simulink model "bldc_motor2"  (Simulink 8.4)
settings: Solver=ode45  StartTime=0.0  StopTime=1  MaxStep=1e-4  RelTol=1e-4  AbsTol=1e-4
values from neighbouring files (symbols this model uses):
  Dm = 6.04e-6    (= 6.04e-06)    [bldc_par.m]
  J = 2.12e-6    (= 2.12e-06)    [bldc_par.m]
  Lam = 0.0165    [bldc_par.m]
  Lss = 10.1e-3    (= 0.0101)    [bldc_par.m]
  P = 2    [bldc_par.m]
  rs = 5.2    [bldc_par.m]
  Tm = 3.53e-3    (= 0.00353)    [bldc_par.m]
  Ts = Lss/rs    (= 0.00194230769231)    [bldc_par.m]
  Vdc = 6    [bldc_par.m]
undefined symbols (not defined in the file or in its folder): sgn
settings Model: Creator=Kevin Ta  LastModifiedBy=Kevin Ta
settings DataIOCC: MaxDataPoints=10000  SaveOutput=off  SaveState=on  StateSaveName=x  TimeSaveName=t  SignalLoggingName=sigsOut
settings OptimizationCC: ExpressionDepthLimit=128  InitFltsAndDblsToZero=on
settings DebuggingCC: SaveWithParameterizedLinksMsg=none  SignalResolutionControl=TryResolveAllWithWarning  SolverPrmCheckMsg=none  MultiTaskDSMMsg=warning  MultiTaskCondExecSysMsg=none  StateNameClashWarn=none
settings HardwareCC: TargetUnknown=on
settings RTWCC: IncludeERTFirstTime=on
settings GRTTargetCC: TargetFcnLib=ansi_tfl_tmw.mat

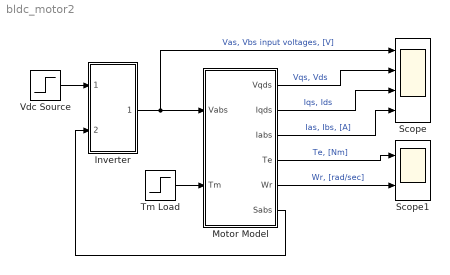
== system bldc_motor2 ==
  Inverter : Subsystem
  Motor Model : Subsystem
  Scope : Scope  NumInputPorts=4
      settings: TimeRange=1  YMin=-10~-10~-1~-1  YMax=10~10~2~2
  Scope1 : Scope  NumInputPorts=2
      settings: TimeRange=1  YMin=0~0  YMax=0.025~400
  Tm Load : Step  Time=0.5  After=Tm  SampleTime=0
  Vdc Source : Step  Time=0.05  After=Vdc  SampleTime=0
  wires:
  Inverter/1(Vabs) -> Scope/1, Motor Model/1(Vabs)  "Vas, Vbs input voltages, [V]"
  Vdc Source/1 -> Inverter/1(Vdc)
  Motor Model/1(Vqds) -> Scope/2  "Vqs, Vds"
  Motor Model/2(Iqds) -> Scope/3  "Iqs, Ids"
  Motor Model/3(Iabs) -> Scope/4  "Ias, Ibs, [A]"
  Motor Model/4(Te) -> Scope1/1  "Te, [Nm]"
  Motor Model/5(Wr) -> Scope1/2  "Wr, [rad/sec]"
  Tm Load/1 -> Motor Model/2(Tm)
  Motor Model/6(Sabs) -> Inverter/2(Sabs)

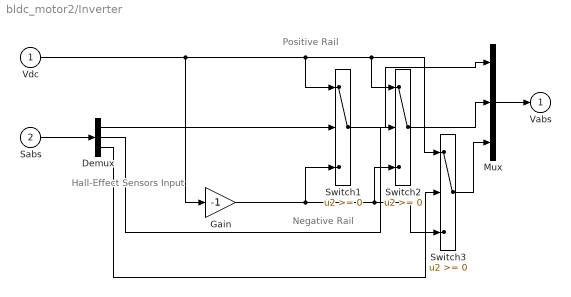
== system bldc_motor2/Inverter ==
  note: Positive Rail
  note: Negative Rail
  note: Hall-Effect
      | Sensors
      | Input
  Vdc : Inport
  Sabs : Inport  Port=2
  Demux : Demux  Outputs=3
  Gain : Gain  Gain=-1  SaturateOnIntegerOverflow=on  OutDataTypeStr=Inherit: Same as input  ParamDataTypeStr=Inherit: Same as input
  Mux : Mux  Inputs=3
  Switch1 : Switch  SaturateOnIntegerOverflow=on
  Switch2 : Switch  SaturateOnIntegerOverflow=on
  Switch3 : Switch  SaturateOnIntegerOverflow=on
  Vabs : Outport  InitialOutput=0
  wires:
  Vdc/1 -> Switch1/1, Switch3/1, Switch2/1, Gain/1
  Gain/1 -> Switch1/3, Switch3/3, Switch2/3
  Switch1/1 -> Mux/1
  Switch2/1 -> Mux/2
  Mux/1 -> Vabs/1
  Sabs/1 -> Demux/1
  Demux/1 -> Switch1/2
  Demux/2 -> Switch2/2
  Demux/3 -> Switch3/2
  Switch3/1 -> Mux/3

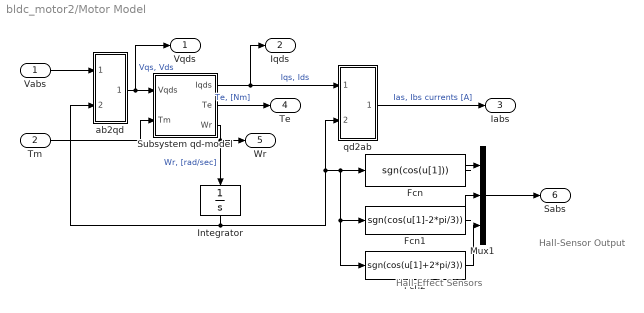
== system bldc_motor2/Motor Model ==
  note: Hall-Effect
      | Sensors
  note: Hall-Sensor
      | Output
  Vabs : Inport
  Tm : Inport  Port=2
  Fcn : Fcn  Expr=sgn(cos(u[1]))
  Fcn1 : Fcn  Expr=sgn(cos(u[1]-2*pi/3))
  Fcn2 : Fcn  Expr=sgn(cos(u[1]+2*pi/3))
  Integrator : Integrator
  Mux1 : Mux  Inputs=3
  Subsystem qd-model : Subsystem
  ab2qd : Subsystem
  qd2ab : Subsystem
  Vqds : Outport
  Iqds : Outport  Port=2
  Iabs : Outport  Port=3
  Te : Outport  Port=4
  Wr : Outport  Port=5
  Sabs : Outport  Port=6
  wires:
  ab2qd/1(Vqds) -> Subsystem qd-model/1(Vqds), Vqds/1  "Vqs, Vds"
  Subsystem qd-model/1(Iqds) -> qd2ab/1(Iqds), Iqds/1  "Iqs, Ids"
  Subsystem qd-model/3(Wr) -> Integrator/1, Wr/1  "Wr, [rad/sec]"
  Integrator/1 -> ab2qd/2(theta), qd2ab/2(theta), Fcn/1, Fcn2/1, Fcn1/1
  Vabs/1 -> ab2qd/1(Vabs)
  Subsystem qd-model/2(Te) -> Te/1  "Te, [Nm]"
  qd2ab/1(Iabs) -> Iabs/1  "Ias, Ibs currents [A]"
  Tm/1 -> Subsystem qd-model/2(Tm)
  Fcn/1 -> Mux1/1
  Fcn1/1 -> Mux1/2
  Mux1/1 -> Sabs/1
  Fcn2/1 -> Mux1/3

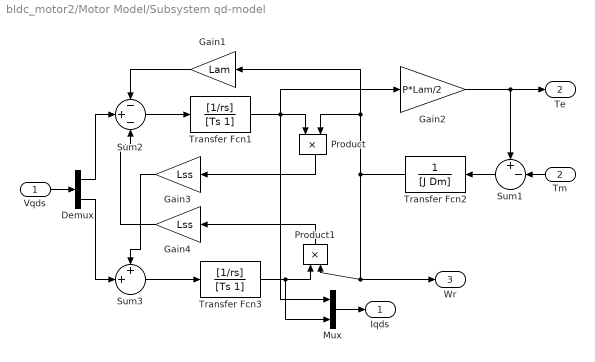
== system bldc_motor2/Motor Model/Subsystem qd-model ==
  Vqds : Inport
  Tm : Inport  Port=2
  Demux : Demux  Outputs=2
  Gain1 : Gain  Gain=Lam  SaturateOnIntegerOverflow=on  OutDataTypeStr=Inherit: Same as input  ParamDataTypeStr=Inherit: Same as input
  Gain2 : Gain  Gain=P*Lam/2  SaturateOnIntegerOverflow=on  OutDataTypeStr=Inherit: Same as input  ParamDataTypeStr=Inherit: Same as input
  Gain3 : Gain  Gain=Lss  SaturateOnIntegerOverflow=on  OutDataTypeStr=Inherit: Same as input  ParamDataTypeStr=Inherit: Same as input
  Gain4 : Gain  Gain=Lss  SaturateOnIntegerOverflow=on  OutDataTypeStr=Inherit: Same as input  ParamDataTypeStr=Inherit: Same as input
  Mux : Mux  Inputs=2
  Product : Product  SaturateOnIntegerOverflow=on  OutDataTypeStr=Inherit: Same as first input
  Product1 : Product  SaturateOnIntegerOverflow=on  OutDataTypeStr=Inherit: Same as first input
  Sum1 : Sum  Inputs=+-|  SaturateOnIntegerOverflow=on
  Sum2 : Sum  Inputs=-+-  SaturateOnIntegerOverflow=on
  Sum3 : Sum  Inputs=++|  SaturateOnIntegerOverflow=on
  Transfer Fcn1 : TransferFcn  Numerator=[1/rs]  Denominator=[Ts 1]
  Transfer Fcn2 : TransferFcn  Denominator=[J Dm]
  Transfer Fcn3 : TransferFcn  Numerator=[1/rs]  Denominator=[Ts 1]
  Iqds : Outport
  Te : Outport  Port=2
  Wr : Outport  Port=3
  wires:
  Sum2/1 -> Transfer Fcn1/1
  Gain1/1 -> Sum2/1
  Transfer Fcn1/1 -> Product/1, Gain2/1, Mux/1
  Transfer Fcn2/1 -> Product/2, Gain1/1, Product1/2, Wr/1
  Sum3/1 -> Transfer Fcn3/1
  Product/1 -> Gain3/1
  Gain3/1 -> Sum3/1
  Transfer Fcn3/1 -> Product1/1, Mux/2
  Gain4/1 -> Sum2/3
  Product1/1 -> Gain4/1
  Sum1/1 -> Transfer Fcn2/1
  Gain2/1 -> Sum1/1, Te/1
  Tm/1 -> Sum1/2
  Demux/1 -> Sum2/2
  Demux/2 -> Sum3/2
  Vqds/1 -> Demux/1
  Mux/1 -> Iqds/1

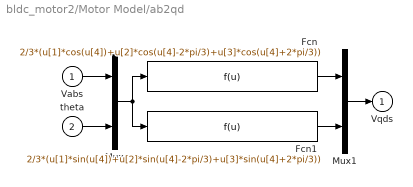
== system bldc_motor2/Motor Model/ab2qd ==
  Vabs : Inport
  theta : Inport  Port=2
  Fcn : Fcn  Expr=2/3*(u[1]*cos(u[4])+u[2]*cos(u[4]-2*pi/3)+u[3]*cos(u[4]+2*pi/3))
  Fcn1 : Fcn  Expr=2/3*(u[1]*sin(u[4])+u[2]*sin(u[4]-2*pi/3)+u[3]*sin(u[4]+2*pi/3))
  Mux : Mux  Inputs=[3,1]
  Mux1 : Mux  Inputs=2
  Vqds : Outport  InitialOutput=0
  wires:
  Mux/1 -> Fcn/1, Fcn1/1
  Mux1/1 -> Vqds/1
  Fcn/1 -> Mux1/1
  Fcn1/1 -> Mux1/2
  Vabs/1 -> Mux/1
  theta/1 -> Mux/2

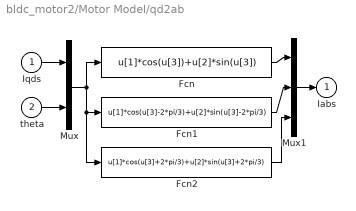
== system bldc_motor2/Motor Model/qd2ab ==
  Iqds : Inport
  theta : Inport  Port=2
  Fcn : Fcn  Expr=u[1]*cos(u[3])+u[2]*sin(u[3])
  Fcn1 : Fcn  Expr=u[1]*cos(u[3]-2*pi/3)+u[2]*sin(u[3]-2*pi/3)
  Fcn2 : Fcn  Expr=u[1]*cos(u[3]+2*pi/3)+u[2]*sin(u[3]+2*pi/3)
  Mux : Mux  Inputs=[2,1]
  Mux1 : Mux  Inputs=3
  Iabs : Outport  InitialOutput=0
  wires:
  Mux/1 -> Fcn/1, Fcn2/1, Fcn1/1
  Mux1/1 -> Iabs/1
  Fcn/1 -> Mux1/1
  Fcn1/1 -> Mux1/2
  Iqds/1 -> Mux/1
  theta/1 -> Mux/2
  Fcn2/1 -> Mux1/3
